simulink model "s4"  (Simulink 2.00)
settings: Solver=ode45  StartTime=0.0  StopTime=tstop  MaxStep=5e-3  RelTol=1e-5  AbsTol=1e-6
values from neighbouring files (symbols this model uses):
  C = 1000e-6    (= 0.001)    [M2.M]    (also in M2INIT.M; M4.M = 1.082251e-07)
  iLo = 0    [M2.M]    (also in M2INIT.M; M3.M; M4.M)
  L = 0.1    [M2.M]    (also in M2INIT.M; M3.M = 0.04; M4.M = 0.000231)
  Pref_time = [ 0 6e-4 11e-4 11e-4 18e-4 18e-4 tstop ]    [M4.M]
  Pref_value = [ 0 600 600 300 300 600 600 ]    [M4.M]
  R = 0.4    [M3.M]    (also in M4.M = 12)
  vCo = 0    [M2.M]    (also in M2INIT.M; M4.M)
  Vdc = 100    [M4.M]
  wo = sqrt(1/(L*C))    [M4.M]
settings Model: SaveTime=off  SaveOutput=off  ConsistencyChecking=off

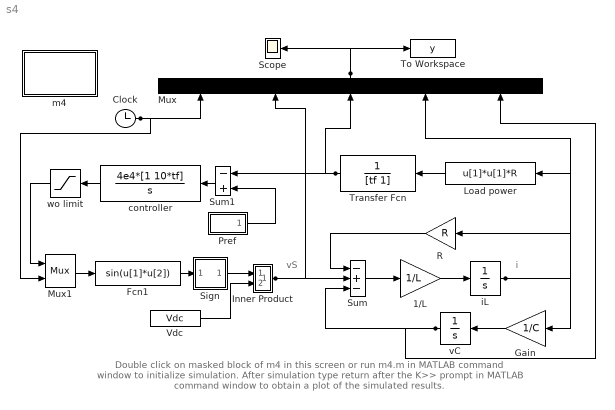
== system s4 ==
  note: i
  note: vS
  note: Double click on masked block of m4 in this screen or run m4.m in MATLAB command window
      | to initialize simulation.  After simulation type return after the K>> prompt in MATLAB command
      | window to obtain a plot of the simulated results.
  1/L : Gain  Gain=1/L
  Clock : Clock
      settings: DeleteFcn=simclock BlockIsBeingDestroyed  PostSaveFcn=simclock Save
  m4 : Subsystem
      settings: OpenFcn=m4
      mask Type: Masked block of m4.m
      mask Help: Uses m4.m to initialize and plot
      mask Display: disp('Initialize\nand plot')
  Fcn1 : Fcn  Expr=sin(u[1]*u[2])
  Gain : Gain  Orientation=left  Gain=1/C
  Inner Product : Subsystem
      mask Type: Dot Product
      mask Description:
      | Inner (dot) product.
      | y=sum(u1.*u2)
      mask Help: Computes the inner (dot) product of the inputs: sum(u1.*u2).  The inputs are vectors of the same length. Output is a scalar.
      mask Display: disp('.\n')
  Load power : Fcn  Orientation=left  Expr=u[1]*u[1]*R
  Mux : Mux  Orientation=up  Inputs=5
  Mux1 : Mux  Inputs=2
  Pref : Subsystem  mask(Repeating table){rep_seq_t=Pref_time, rep_seq_y=Pref_value}
      mask prompts: rep_seq_t "Time values:"; rep_seq_y "Output values:"
      mask help: Repeating table.
      mask init:
      | period = max(rep_seq_t);
      mask Help: Repeats cycle given in table. Time values should be monotonically increasing.
      mask Display: plot([rep_seq_t,rep_seq_t+period,rep_seq_t+2*period,rep_seq_t(1)+3*period],[rep_seq_y,rep_seq_y,rep_seq_y,rep_seq_y(1)])
  R : Gain  Orientation=left  Gain=R
  Scope : Scope
      settings: TickLabels=on  TimeRange=auto  YMin=-600  YMax=600  SaveToWorkspace=off  SaveName=ScopeData
  Sign : Subsystem
      mask Type: Sign
      mask Description: y = sign(x)
      mask Help: Sign Function:\n\t\t\ty = 1 if x > 0\n\t\t\ty = 0 if x = 0\n\t\t\ty = -1 if x < 0
      mask Display: plot(-50,-50,50,50,[-50,50],[0,0],[0,0],[-50,50],[-40,0],[-30,-30],[0,40],[30,30])
  Sum : Sum  Inputs=-+-
  Sum1 : Sum  Orientation=left  Inputs=-+
  To Workspace : ToWorkspace  VariableName=y  SampleTime=0
      settings: Buffer=100000
  Transfer Fcn : TransferFcn  Orientation=left  Numerator=[1]  Denominator=[tf 1]
  Vdc : Constant  Value=Vdc
  controller : TransferFcn  Orientation=left  Numerator=4e4*[1 10*tf]  Denominator=[1 0]
  iL : Integrator  ExternalReset=none  InitialConditionSource=internal  InitialCondition=iLo  LimitOutput=off  UpperSaturationLimit=inf  LowerSaturationLimit=-inf  ShowSaturationPort=off  ShowStatePort=off  AbsoluteTolerance=auto
  vC : Integrator  Orientation=left  ExternalReset=none  InitialConditionSource=internal  InitialCondition=vCo  LimitOutput=off  UpperSaturationLimit=inf  LowerSaturationLimit=-inf  ShowSaturationPort=off  ShowStatePort=off  AbsoluteTolerance=auto
  wo limit : Saturate  Orientation=left  UpperLimit=wo  LowerLimit=0
  wires:
  Pref/1(out_1) -> Sum1/2
  controller/1 -> wo limit/1
  Transfer Fcn/1 -> Mux/3, Sum1/1
  wo limit/1 -> Mux1/1
  Clock/1 -> Mux1/2, Mux/1
  Mux1/1 -> Fcn1/1
  vC/1 -> Mux/5, Sum/3
  Inner Product/1(out_1) -> Mux/2, Sum/2
  Sign/1(out_1) -> Inner Product/1(in_1)
  Vdc/1 -> Inner Product/2(in_2)
  Fcn1/1 -> Sign/1(in_1)
  Sum1/1 -> controller/1
  Load power/1 -> Transfer Fcn/1
  Gain/1 -> vC/1
  iL/1 -> Mux/4, Load power/1, Gain/1, R/1
  R/1 -> Sum/1
  Sum/1 -> 1/L/1
  Mux/1 -> Scope/1, To Workspace/1
  1/L/1 -> iL/1

== system s4/m4 ==
  note: Masked block of m4.m to initialize
      | and plot results

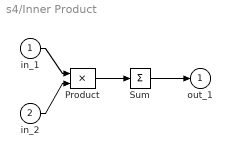
== system s4/Inner Product ==
  in_1 : Inport  Port=1  PortWidth=-1  SampleTime=-1
  in_2 : Inport  Port=2  PortWidth=-1  SampleTime=-1
  Product : Product  Inputs=2
  Sum : Sum  Inputs=+
  out_1 : Outport  Port=1  InitialOutput=0
  wires:
  Sum/1 -> out_1/1
  Product/1 -> Sum/1
  in_1/1 -> Product/1
  in_2/1 -> Product/2

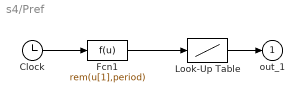
== system s4/Pref ==
  Clock : Clock
      settings: DeleteFcn=simclock BlockIsBeingDestroyed  PostSaveFcn=simclock Save
  Fcn1 : Fcn  Expr=rem(u[1],period)
  Look-Up Table : Lookup  InputValues=rep_seq_t  OutputValues=rep_seq_y
  out_1 : Outport  Port=1  InitialOutput=0
  wires:
  Fcn1/1 -> Look-Up Table/1
  Clock/1 -> Fcn1/1
  Look-Up Table/1 -> out_1/1

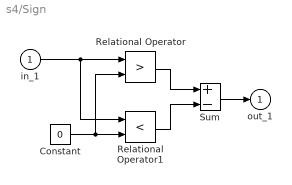
== system s4/Sign ==
  in_1 : Inport  Port=1  PortWidth=-1  SampleTime=-1
  Constant : Constant  Value=0
  Relational Operator : RelationalOperator  Operator=>
  Relational Operator1 : RelationalOperator  Operator=<
  Sum : Sum  Inputs=+-
  out_1 : Outport  Port=1  InitialOutput=0
  wires:
  Sum/1 -> out_1/1
  Relational Operator/1 -> Sum/1
  Relational Operator1/1 -> Sum/2
  Constant/1 -> Relational Operator/2, Relational Operator1/2
  in_1/1 -> Relational Operator1/1, Relational Operator/1
